simulink model "ANS_GFM_short_term"  (R2021b)
settings: Solver=FixedStepAuto  StartTime=0.0  StopTime=5  FixedStep=Ts  MaxStep=1e-5  RelTol=1e-3
values from neighbouring files (symbols this model uses):
  angle_load = angle(LF.bus(ind_l).Vbus)*180/pi    [init_ANS_GFM_long_term.m]    (also in init_ANS_GFM_short_term.m)
  angleV_LF = Vangle_init/180*pi    [init_ANS_GFM_long_term.m]    (also in init_ANS_GFM_short_term.m)
  awu = 1    [init_ANS_GFM_long_term.m]    (also in init_ANS_GFM_short_term.m)
  C_dc = 1/(Xcdc_pu_or*Zbase_dc_new*100*pi)    [init_ANS_GFM_long_term.m]    (also in init_ANS_GFM_short_term.m)
  C_f = 1/(Xcf_pu_or*Zbase_new*100*pi)    (= 0.013712)    [init_ANS_GFM_long_term.m]    (also in init_ANS_GFM_short_term.m = 0.0141333333333)
  control = 3    [init_ANS_GFM_long_term.m]    (also in init_ANS_GFM_short_term.m = 1)
  D_p = (1/(m_p*w_b))    (= 5209935.26289)    [init_ANS_GFM_long_term.m]    (also in init_ANS_GFM_short_term.m = 5370022.73304)
  Egrid_tmp = 1.054080675694902*400e3    (= 421632.270278)    [init_ANS_GFM_long_term.m]    (also in init_ANS_GFM_short_term.m)
  epsi = 1e-4    (= 0.0001)    [init_ANS_GFM_long_term.m]    (also in init_ANS_GFM_short_term.m)
  eta = m_p*V_m^2    [init_ANS_GFM_long_term.m]    (also in init_ANS_GFM_short_term.m)
  gamma = 2.3    [init_ANS_GFM_long_term.m]    (also in init_ANS_GFM_short_term.m)
  I0_init = [I0_init_a, I0_init_b, I0_init_c]    [init_ANS_GFM_long_term.m]    (also in init_ANS_GFM_short_term.m)
  I_bc = S_bc / (V_bc*sqrt(3))    [init_ANS_GFM_long_term.m]    (also in init_ANS_GFM_short_term.m)
  I_d_int_init = (U_d_int + I_q_int*L_f*w_b - V_d_int - I_d_int*R_f*0)    [init_ANS_GFM_long_term.m]    (also in init_ANS_GFM_short_term.m)
  I_init = [I_init_a, I_init_b, I_init_c]    [init_ANS_GFM_long_term.m]    (also in init_ANS_GFM_short_term.m)
  i_ll = -1.15*(S_bc/Vdc_n)-i_loss_dc    [init_ANS_GFM_long_term.m]    (also in init_ANS_GFM_short_term.m)
  I_max_sat_pu = 1.0 * I_bc *sqrt(2)    [init_ANS_GFM_long_term.m]    (also in init_ANS_GFM_short_term.m)
  I_q_int_init = (U_q_int - I_d_int*L_f*w_b - V_q_int - I_q_int*R_f*0)    [init_ANS_GFM_long_term.m]    (also in init_ANS_GFM_short_term.m)
  i_ul = 1.15*(S_bc/Vdc_n)+i_loss_dc    [init_ANS_GFM_long_term.m]    (also in init_ANS_GFM_short_term.m)
  idppu = 0.95    [init_ANS_GFM_long_term.m]    (also in init_ANS_GFM_short_term.m = 0.92)
  init_dP = -inv(A_pm)*B_pm*dP    [init_ANS_GFM_long_term.m]    (also in init_ANS_GFM_short_term.m)
  init_pm = -inv(A_pm)*B_pm*P_aft    [init_ANS_GFM_long_term.m]    (also in init_ANS_GFM_short_term.m)
  init_tau = -inv(A_tau)*B_tau*idc    [init_ANS_GFM_long_term.m]    (also in init_ANS_GFM_short_term.m)
  J = D_p*tau_f    (= 104198.705258)    [init_ANS_GFM_long_term.m]    (also in init_ANS_GFM_short_term.m = 107400.454661)
  k_dc = eta_1/(Vdc_n*m_p)    [init_ANS_GFM_long_term.m]    (also in init_ANS_GFM_short_term.m)
  K_p = (1/Vdc_n)    [init_ANS_GFM_long_term.m]    (also in init_ANS_GFM_short_term.m)
  K_r = 1/R_dc    [init_ANS_GFM_long_term.m]    (also in init_ANS_GFM_short_term.m)
  Kff_i = 1    [init_ANS_GFM_long_term.m]    (also in init_ANS_GFM_short_term.m)
  Kff_v = 1    [init_ANS_GFM_long_term.m]    (also in init_ANS_GFM_short_term.m)
  Ki_i = (1/n)*1.19    (= 0.0520711785298)    [init_ANS_GFM_long_term.m]    (also in init_ANS_GFM_short_term.m = 0.0505188679245)
  Ki_pll = 4255.3    [init_ANS_GFM_long_term.m]    (also in init_ANS_GFM_short_term.m)
  Ki_v = (n)*1.161022    (= 26.5332227733)    [init_ANS_GFM_long_term.m]    (also in init_ANS_GFM_short_term.m = 27.3485182222)
  ki_v_ac = 2*0.25    (= 0.5)    [init_ANS_GFM_long_term.m]    (also in init_ANS_GFM_short_term.m)
  Kp_i = 0.738891/n    (= 0.032331869895)    [init_ANS_GFM_long_term.m]    (also in init_ANS_GFM_short_term.m = 0.0313680141509)
  Kp_pll = 92    [init_ANS_GFM_long_term.m]    (also in init_ANS_GFM_short_term.m)
  Kp_v = 0.52*n    (= 11.8837333333)    [init_ANS_GFM_long_term.m]    (also in init_ANS_GFM_short_term.m = 12.2488888889)
  kp_v_ac = 0.001    [init_ANS_GFM_long_term.m]    (also in init_ANS_GFM_short_term.m)
  Kpl = 5.0    (= 5)    [init_ANS_GFM_long_term.m]    (also in init_ANS_GFM_short_term.m)
  L1 = cf/sqrt(1+RX^2)*(400e3)^2/Skss/(100*pi)    [init_ANS_GFM_long_term.m]    (also in init_ANS_GFM_short_term.m)
  L_f = Xlf_pu_or*Zbase_new/100/pi    (= 4.37572928821e-06)    [init_ANS_GFM_long_term.m]    (also in init_ANS_GFM_short_term.m = 4.24528301887e-06)
  Lf = 1e6/100/pi    (= 3183.09886184)    [init_ANS_GFM_long_term.m]    (also in init_ANS_GFM_short_term.m = 0.0636619772368)
  m_p = (2*pi*0.5)/(S_bc)    (= 6.10967066042e-10)    [init_ANS_GFM_long_term.m]    (also in init_ANS_GFM_short_term.m = 5.92753330866e-10)
  n = 1/Zb    (= 22.8533333333)    [init_ANS_GFM_long_term.m]    (also in init_ANS_GFM_short_term.m = 23.5555555556)
  P_LF_si = P_LF*S_b    [init_ANS_GFM_long_term.m]    (also in init_ANS_GFM_short_term.m)
  ps = 4440e6/S_bc    (= 0.863477246208)    [init_ANS_GFM_long_term.m]    (also in init_ANS_GFM_short_term.m = 0.837735849057)
  Q_LF_si = Q_LF*S_b    [init_ANS_GFM_long_term.m]    (also in init_ANS_GFM_short_term.m)
  qs = Q_LF*S_b/S_bc    [init_ANS_GFM_long_term.m]    (also in init_ANS_GFM_short_term.m)
  R1 = RX*cf/sqrt(1+RX^2)*(400e3)^2/Skss    [init_ANS_GFM_long_term.m]    (also in init_ANS_GFM_short_term.m)
  R_dc = Rdc_pu_or*Zbase_dc_new    [init_ANS_GFM_long_term.m]    (also in init_ANS_GFM_short_term.m)
  R_f = Rf_pu_or*Zbase_new    (= 2.18786464411e-05)    [init_ANS_GFM_long_term.m]    (also in init_ANS_GFM_short_term.m = 2.12264150943e-05)
  Rf = 1e6    (= 1000000)    [init_ANS_GFM_long_term.m]    (also in init_ANS_GFM_short_term.m = 20)
  S_bc = 5142e6    (= 5142000000)    [init_ANS_GFM_long_term.m]    (also in init_ANS_GFM_short_term.m = 5300000000)
  sat_select = 3    [init_ANS_GFM_long_term.m]    (also in init_ANS_GFM_short_term.m)
  SECM = 3    [init_ANS_GFM_long_term.m]    (also in init_ANS_GFM_short_term.m = 1)
  share_i_load = 1.0    (= 1)    [init_ANS_GFM_long_term.m]    (also in init_ANS_GFM_short_term.m)
  T_en = -0.5    [init_ANS_GFM_long_term.m]    (also in init_ANS_GFM_short_term.m)
  T_off = T_on + 0.1    (= 0.2)    [init_ANS_GFM_long_term.m]    (also in init_ANS_GFM_short_term.m)
  T_on = 0.1    [init_ANS_GFM_long_term.m]    (also in init_ANS_GFM_short_term.m)
  Ts = 2e-6    (= 2e-06)    [init_ANS_GFM_long_term.m]    (also in init_ANS_GFM_short_term.m = 1e-06)
  U_init = [Umag_init_a, Umag_init_b, Umag_init_c]    [init_ANS_GFM_long_term.m]    (also in init_ANS_GFM_short_term.m)
  Uangle_init = angle(V_LF_VSC)*180/pi    [init_ANS_GFM_long_term.m]    (also in init_ANS_GFM_short_term.m)
  Umag_init = abs(V_LF_VSC)*V_bc*sqrt(2/3)    [init_ANS_GFM_long_term.m]    (also in init_ANS_GFM_short_term.m)
  V1_rms = 15e3    (= 15000)    [init_ANS_GFM_long_term.m]    (also in init_ANS_GFM_short_term.m)
  V_d_int = abs(V_LF)*V_bc*sqrt(2/3)    [init_ANS_GFM_long_term.m]    (also in init_ANS_GFM_short_term.m)
  V_d_int_init = (I_d_int + V_q_int*C_f*w_b - I0_d_int)    [init_ANS_GFM_long_term.m]    (also in init_ANS_GFM_short_term.m)
  V_init = [V_init_a, V_init_b, V_init_c]    [init_ANS_GFM_long_term.m]    (also in init_ANS_GFM_short_term.m)
  V_m = sqrt(2/3)*V_bc    [init_ANS_GFM_long_term.m]    (also in init_ANS_GFM_short_term.m)
  V_q_int_init = (I_q_int - V_d_int*C_f*w_b - I0_q_int)    [init_ANS_GFM_long_term.m]    (also in init_ANS_GFM_short_term.m)
  Vdc_n = 3*V_m    [init_ANS_GFM_long_term.m]    (also in init_ANS_GFM_short_term.m)
  Vref = V_LF_mag*V_m    [init_ANS_GFM_long_term.m]    (also in init_ANS_GFM_short_term.m)
  w_b = 2*pi*f_b    (= 314.159265359)    [init_ANS_GFM_long_term.m]    (also in init_ANS_GFM_short_term.m)
  w_f = 2*pi*5    (= 31.4159265359)    [init_ANS_GFM_long_term.m]    (also in init_ANS_GFM_short_term.m)
  Zbase_new = V1_rms^2/S_bc    (= 0.0437572928821)    [init_ANS_GFM_long_term.m]    (also in init_ANS_GFM_short_term.m = 0.0424528301887)
undefined symbols (not defined in the file or in its folder): A_pm, A_tau, B_pm, B_tau, C_pm, C_tau, D_pm, D_tau, find_system, idq0_init, Pm, sm_init, v_d, v_q, Ve
libraries: spsBreakerLib x270, spsGroundLib x21, spsThreePhaseSeriesRLCBranchLib x12, spsabctodq0Lib x11, simulink x9, spsEdgeDetectorLib x8, spsThreePhaseVIMeasurementLib x7, spsLoadFlowBusLib x7, spsSeriesRLCBranchLib x6, spsControlledVoltageSourceLib x6, spsCurrentMeasurementLib x6, spsVoltageMeasurementLib x6
(part 2 of 7)

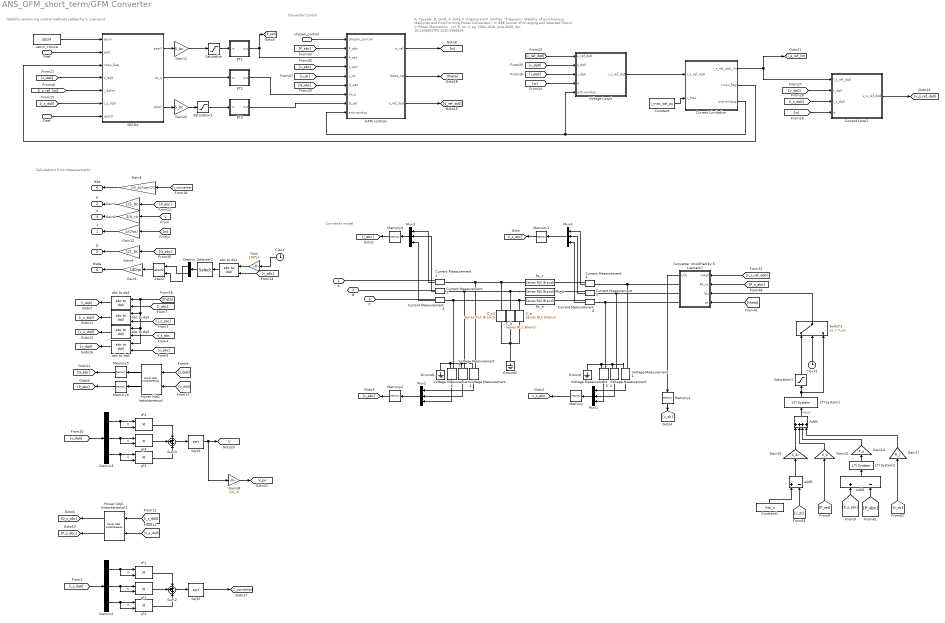
== system ANS_GFM_short_term/GFM Converter ==
  note: A. Tayyebi, D. Groß, A. Anta, F. Kupzog and F. Dörfler, "Frequency Stability of Synchronous Machines and Grid-Forming Power Converters," in IEEE Journal of Emerging and Selected Topics in Power Electronics , vol. 8, no. 2, pp. 1004-1018, June 2020, doi: 10.1109/JESTPE.2020.2966524.
  note: Calculations from Measurements
  note: Converter Control
  note: Stability-enhancing control methods (added by S. Liemann)
  note: Converter model
  chosen_control : Inport
  Pset : Inport  Port=2
  Qset : Inport  Port=3
  Add2 : Sum  Inputs=+-
  Add4 : Sum  Inputs=++++
  Add6 : Sum  Inputs=+-
  Atan2 : Trigonometry  Operator=atan2
  C_a : spsSeriesRLCBranchLib/Series RLC Branch  LConnTagsString=__new0  RConnTagsString=__new0  BranchType=C  Resistance=1  Inductance=1e-3  SetiL0=off  InitialCurrent=0  Capacitance=C_f  Setx0=on  InitialVoltage=V_init_c  Measurements=None
  C_b : spsSeriesRLCBranchLib/Series RLC Branch  LConnTagsString=__new0  RConnTagsString=__new0  BranchType=C  Resistance=1  Inductance=1e-3  SetiL0=off  InitialCurrent=0  Capacitance=C_f  Setx0=on  InitialVoltage=V_init_b  Measurements=None
  C_c1 : spsSeriesRLCBranchLib/Series RLC Branch  LConnTagsString=__new0  RConnTagsString=__new0  BranchType=C  Resistance=1  Inductance=1e-3  SetiL0=off  InitialCurrent=0  Capacitance=C_f  Setx0=on  InitialVoltage=V_init_a  Measurements=None
  Clock : Clock
  Clock1 : Clock
  Constant : Constant  Value=I_max_sat_pu
  Constant1 : Constant  Value=Vdc_n
  Converter (modified by S. Liemann) : Subsystem
  Current Limitation : Subsystem
  Current Loop1 : Subsystem
  Current Measurement{1..6} (6 alike) : spsCurrentMeasurementLib/Current Measurement  PhasorSimulation=off  OutputType=Complex  PSBequivalent=0
  Demux : Demux  Outputs=2
  Demux2 : Demux  Outputs=3
  Demux3 : Demux  Outputs=3
  GFM controls : Subsystem
  Gain : Gain  Gain=100*pi
  Gain1 : Gain  Gain=180/pi
  Gain11 : Gain  Gain=S_bc
  Gain12 : Gain  Gain=1/(2*pi)
  Gain13 : Gain  Gain=K_p
  Gain14 : Gain  Gain=K_p
  Gain16 : Gain  Gain=k_dc
  Gain17 : Gain  Gain=K_r
  Gain18 : Gain  Gain=1/V_m
  Gain22 : Gain  Gain=S_bc
  Gain3 : Gain  Gain=1/(I_bc*sqrt(2))
  Gain4 : Gain  Gain=1/S_bc
  Gain6 : Gain  Gain=1/V_m
  Gain7 : Gain  Gain=1/S_bc
  Ground : spsGroundLib/Ground  LConnTagsString=a
  Ground1 : spsGroundLib/Ground  LConnTagsString=a
  Ground2 : spsGroundLib/Ground  LConnTagsString=a
  LTI System1 : cstblocks/LTI System  sys=ss(A_tau,B_tau,C_tau,D_tau)  IC=[init_tau]
  LTI System2 : cstblocks/LTI System  sys=ss(A_pm,B_pm,C_pm,D_pm)  IC=[init_dP]
  Memory : Memory  InitialCondition=U_init
  Memory1 : Memory  InitialCondition=I_init
  Memory2 : Memory  InitialCondition=V_init
  Memory3 : Memory  InitialCondition=I0_init
  Memory4 : Memory  InitialCondition=Vdc_n
  Memory5 : Memory  InitialCondition=Q_LF_si
  Memory6 : Memory  InitialCondition=P_LF_si
  Mux{1..4} (4 alike) : Mux  Inputs=3
  PT1 : Subsystem
  PT2 : Subsystem
  PT3 : Subsystem
  "Power (dq0, Instantaneous)" : spsPowerdq0InstantaneousLib/Power (dq0, Instantaneous)
      settings: SourceProductBaseCode=PS
  "Power (dq0, Instantaneous)1" : spsPowerdq0InstantaneousLib/Power (dq0, Instantaneous)
      settings: SourceProductBaseCode=PS
  RL_a : spsSeriesRLCBranchLib/Series RLC Branch  LConnTagsString=__new0  RConnTagsString=__new0  BranchType=RL  Resistance=R_f  Inductance=L_f  SetiL0=on  InitialCurrent=I_init_c  Capacitance=1e-6  Setx0=off  InitialVoltage=0  Measurements=Branch voltage and current
  RL_b : spsSeriesRLCBranchLib/Series RLC Branch  LConnTagsString=__new0  RConnTagsString=__new0  BranchType=RL  Resistance=R_f  Inductance=L_f  SetiL0=on  InitialCurrent=I_init_b  Capacitance=1e-6  Setx0=off  InitialVoltage=0  Measurements=None
  RL_c : spsSeriesRLCBranchLib/Series RLC Branch  LConnTagsString=__new0  RConnTagsString=__new0  BranchType=RL  Resistance=R_f  Inductance=L_f  SetiL0=on  InitialCurrent=I_init_a  Capacitance=1e-6  Setx0=off  InitialVoltage=0  Measurements=None
  SECMs : Subsystem
  Saturation : Saturate  UpperLimit=S_bc  LowerLimit=-S_bc
  Saturation1 : Saturate  UpperLimit=i_ul  LowerLimit=i_ll
  Saturation2 : Saturate  UpperLimit=S_bc  LowerLimit=-S_bc
  Selector2 : Selector  InputPortWidth=3  IndexOptions=Index vector (dialog)  Indices=[1 2]  OutputSizes=1
  Sqrt2 : Sqrt  SaturateOnIntegerOverflow=on
  Sqrt3 : Sqrt  SaturateOnIntegerOverflow=on
  Sum2 : Sum  Inputs=+++  InputSameDT=on  SaturateOnIntegerOverflow=on  OutDataTypeStr=Inherit: Same as first input
  Sum3 : Sum  Inputs=+++  InputSameDT=on  SaturateOnIntegerOverflow=on  OutDataTypeStr=Inherit: Same as first input
  Switch1 : Switch  Criteria=u2 > Threshold  Threshold=T_en
  Voltage Loop1 : Subsystem
  Voltage Measurement{1..6} (6 alike) : spsVoltageMeasurementLib/Voltage Measurement  PhasorSimulation=off  OutputType=Complex  PSBequivalent=0
  abc to dq{1,3..6} (5 alike) : spsabctodq0Lib/abc to dq0  Alignment=90 degrees behind phase A axis
  d²1 : Product  InputSameDT=on  RndMeth=Zero  SaturateOnIntegerOverflow=on  OutDataTypeStr=Inherit: Same as first input
  d²2 : Product  InputSameDT=on  RndMeth=Zero  SaturateOnIntegerOverflow=on  OutDataTypeStr=Inherit: Same as first input
  q²{1..2,4..5} (4 alike) : Product  InputSameDT=on  RndMeth=Zero  SaturateOnIntegerOverflow=on  OutDataTypeStr=Inherit: Same as first input
  secm_choice : Constant  Value=SECM
  A : PMIOPort  Side=Right
  B : PMIOPort  Port=2  Side=Right
  C : PMIOPort  Port=3  Side=Right
  f : Outport  VectorParamsAs1DForOutWhenUnconnected=off
  P : Outport  Port=2  VectorParamsAs1DForOutWhenUnconnected=off
  V : Outport  Port=3  VectorParamsAs1DForOutWhenUnconnected=off
  Iabs : Outport  Port=4  VectorParamsAs1DForOutWhenUnconnected=off
  Q : Outport  Port=5  VectorParamsAs1DForOutWhenUnconnected=off
  theta : Outport  Port=6  VectorParamsAs1DForOutWhenUnconnected=off
  tag scope: V=global, V_pu=global, v_s_abc=global
  wires:
  [i_s_dq0] -> "Power (dq0, Instantaneous)1"/2
  Voltage Measurement5/1 -> Mux2/2
  [v_s_dq0] -> "Power (dq0, Instantaneous)1"/1
  Voltage Measurement3/1 -> Mux1/3
  Voltage Measurement1/1 -> Mux1/1
  Memory1/1 -> [i_s_abc]
  q²1/1 -> Sum2/2
  Current Measurement4/1 -> Mux4/1
  Mux3/1 -> Memory3/1
  Constant1/1 -> Add6/1
  Voltage Measurement4/1 -> Mux2/1
  [I_converter] -> Gain3/1
  LTI System1/1 -> Saturation1/1, Switch1/3
  Memory2/1 -> [v_abc]
  Memory/1 -> [v_s_abc]
  Sum2/1 -> Sqrt2/1
  Demux2/2 -> q²1/2, q²1/1  "q"
  Add6/1 -> Gain16/1
  [v_dq0] -> "Power (dq0, Instantaneous)"/1
  Current Measurement5/1 -> Mux4/2
  Gain3/1 -> Iabs/1
  [i_s_dq0] -> Demux2/1
  [theta] -> abc to dq3/2, abc to dq6/2, abc to dq5/2, abc to dq4/2
  d²1/1 -> Sum2/1
  [P_abc] -> Gain7/1
  Voltage Measurement2/1 -> Mux1/2
  [P_s_abc] -> Add2/1
  Demux2/3 -> q²2/2, q²2/1  "0"
  Gain16/1 -> Add4/1
  Gain13/1 -> Add4/2
  Demux3/2 -> q²4/2, q²4/1  "q"
  "Power (dq0, Instantaneous)1"/2 -> [Q_s_abc]
  Sqrt3/1 -> Gain18/1, [V]
  [P_abc] -> Add2/2
  Saturation1/1 -> Switch1/1
  [v_dc] -> Add6/2
  Demux3/1 -> d²2/2, d²2/1  "d"
  Demux2/1 -> d²1/2, d²1/1  "d"
  [i_abc] -> abc to dq3/1
  Clock1/1 -> Switch1/2
  Current Measurement1/1 -> Mux3/1
  [P_set] -> Gain13/1
  abc to dq4/1 -> [i_s_dq0]
  Add4/1 -> LTI System1/1  "input"
  Current Measurement3/1 -> Mux3/3
  [v_dq0] -> Demux3/1
  Add2/1 -> LTI System2/1
  abc to dq3/1 -> [i_dq0]
  Current Measurement6/1 -> Mux4/3
  Voltage Measurement6/1 -> Mux2/3
  Mux1/1 -> Memory/1
  [v_dc] -> Gain17/1
  [w] -> Gain12/1
  [i_dq0] -> "Power (dq0, Instantaneous)"/2
  Gain12/1 -> f/1
  Gain7/1 -> P/1
  Current Measurement2/1 -> Mux3/2
  [i_s_abc] -> abc to dq4/1
  q²4/1 -> Sum3/2
  Mux2/1 -> Memory2/1
  abc to dq6/1 -> [v_dq0]
  [v_abc] -> abc to dq6/1
  Gain6/1 -> V/1
  [v_s_abc] -> abc to dq5/1
  q²5/1 -> Sum3/3
  Memory3/1 -> [i_abc]
  Memory4/1 -> [v_dc]
  [V] -> Gain6/1
  d²2/1 -> Sum3/1
  Sum3/1 -> Sqrt3/1
  Switch1/1 -> Converter (modified by S. Liemann)/3(Idc)
  q²2/1 -> Sum2/3
  Demux3/3 -> q²5/2, q²5/1  "0"
  Current Limitation/1(i_s_ref_dq0_lim) -> Current Loop1/1(i_s_ref_dq0), [i_s_ref_lim]
  Voltage Loop1/1(i_s_ref_dq0) -> Current Limitation/1(i_s_ref_dq0)
  [i_s_dq0] -> Current Loop1/3(i_s_dq0)
  Current Limitation/3(anti-windup) -> Voltage Loop1/5(anti-windup), GFM controls/9(anti-windup)
  [i_dq0] -> Voltage Loop1/3(i_dq0)
  [w] -> Current Loop1/4(w)
  Constant/1 -> Current Limitation/2(i_max)
  Current Loop1/1(v_s_ref_dq0) -> [v_s_ref_dq0]
  [v_ref_dq0] -> Voltage Loop1/1(v_ref_dq0)
  [v_dq0] -> Current Loop1/2(v_dq0)
  [w] -> Voltage Loop1/4(w)
  Gain4/1 -> Q/1
  [Q_abc] -> Gain4/1
  GFM controls/2(theta_ref) -> [theta]
  GFM controls/3(v_ref_dqo) -> [v_ref_dq0]
  [P_abc] -> GFM controls/2(P_abc)
  PT1/1(out) -> GFM controls/3(P_set), [P_set]
  [v_abc] -> GFM controls/4(v_abc)
  [Q_abc] -> GFM controls/6(Q_abc)
  [v_dc] -> GFM controls/5(v_dc)
  Mux4/1 -> Memory1/1
  [v_dq0] -> Voltage Loop1/2(v_dq0)
  abc to dq5/1 -> [v_s_dq0]
  [v_s_ref_dq0] -> Converter (modified by S. Liemann)/1(Vdq0)
  GFM controls/1(w_ref) -> [w]
  Pset/1 -> SECMs/2(pset)
  [theta] -> Converter (modified by S. Liemann)/4(wt)
  [P_s_abc] -> Converter (modified by S. Liemann)/2(Pe_ac)
  LTI System2/1 -> Gain14/1
  "Power (dq0, Instantaneous)1"/1 -> [P_s_abc]
  "Power (dq0, Instantaneous)"/1 -> Memory6/1
  "Power (dq0, Instantaneous)"/2 -> Memory5/1
  Saturation/1 -> PT1/1(in)
  Memory5/1 -> [Q_abc]
  Memory6/1 -> [P_abc]
  Selector2/1 -> Demux/1
  abc to dq1/1 -> Selector2/1
  Demux/2 -> Atan2/1
  Demux/1 -> Atan2/2
  Atan2/1 -> Gain1/1
  Gain1/1 -> theta/1
  [v_abc] -> abc to dq1/1
  Gain/1 -> abc to dq1/2
  Clock/1 -> Gain/1
  Sqrt2/1 -> [I_converter]
  chosen_control/1 -> GFM controls/1(chosen_control)
  Gain14/1 -> Add4/3
  Gain17/1 -> Add4/4
  Converter (modified by S. Liemann)/1(Udc) -> Memory4/1
  Gain18/1 -> [V_pu]
  [i_s_dq0] -> SECMs/6(i_s_dq0)
  secm_choice/1 -> SECMs/1(secm)
  [v_dq0] -> SECMs/4(V_dq0)
  SECMs/1(pset*) -> Gain11/1
  Gain11/1 -> Saturation/1
  SECMs/2(dv_q) -> PT2/1(in)
  PT2/1(out) -> GFM controls/7(dv_q)
  [i_s_ref_lim] -> SECMs/5(i_dqlim)
  Qset/1 -> SECMs/7(qset0)
  PT3/1(out) -> GFM controls/8(Q_set)
  SECMs/3(qset*) -> Gain22/1
  Gain22/1 -> Saturation2/1
  Saturation2/1 -> PT3/1(in)
  Current Limitation/2(imax_flag) -> SECMs/3(imax_flag)
  connections:
  Ground/LConn1 -- Voltage Measurement3/LConn2 -- Voltage Measurement1/LConn2 -- Voltage Measurement2/LConn2
  Voltage Measurement6/LConn1 -- Current Measurement3/LConn1 -- C_a/LConn1 -- RL_a/RConn1
  Voltage Measurement6/LConn2 -- Ground1/LConn1 -- Voltage Measurement4/LConn2 -- Voltage Measurement5/LConn2
  Voltage Measurement2/LConn1 -- Current Measurement5/LConn1 -- Converter (modified by S. Liemann)/RConn2
  Voltage Measurement4/LConn1 -- Current Measurement1/LConn1 -- C_c1/LConn1 -- RL_c/RConn1
  RL_b/RConn1 -- C_b/LConn1 -- Current Measurement2/LConn1 -- Voltage Measurement5/LConn1
  C_b/RConn1 -- C_c1/RConn1 -- Ground2/LConn1 -- C_a/RConn1
  Current Measurement6/LConn1 -- Voltage Measurement3/LConn1 -- Converter (modified by S. Liemann)/RConn3
  Voltage Measurement1/LConn1 -- Current Measurement4/LConn1 -- Converter (modified by S. Liemann)/RConn1
  Current Measurement4/RConn1 -- RL_c/LConn1
  Current Measurement6/RConn1 -- RL_a/LConn1
  Current Measurement5/RConn1 -- RL_b/LConn1
  Current Measurement1/RConn1 -- A/RConn1
  Current Measurement2/RConn1 -- B/RConn1
  Current Measurement3/RConn1 -- C/RConn1

== system ANS_GFM_short_term/HVRT & LVRT ==
  Uin : Inport
  Clock2 : Clock
  Constant5 : Constant  Value=0
  Constant6 : Constant
  Constant7 : Constant  Value=1.3
  Constant8 : Constant  Value=1.2
  Gain5 : Gain  Gain=0.85/2.85
  Integrator : Integrator
  Relational Operator : RelationalOperator  Operator=<  OutDataTypeStr=boolean  RndMeth=Simplest
  Relational Operator1 : RelationalOperator  Operator=>  OutDataTypeStr=boolean  RndMeth=Simplest
  Switch : Switch  Threshold=T_on+0.15
  Switch1 : Switch  Threshold=T_on+3.0
  Switch2 : Switch  Threshold=T_on+0.1
  HVRT-Flag : Outport
  HVRT curve : Outport  Port=2
  LVRT-Flag : Outport  Port=3
  LVRT curve : Outport  Port=4
  wires:
  Constant5/1 -> Switch/3, Switch1/1
  Integrator/1 -> LVRT curve/1, Relational Operator/2
  Switch2/1 -> HVRT curve/1, Relational Operator1/2
  Relational Operator/1 -> LVRT-Flag/1
  Clock2/1 -> Switch2/2, Switch/2, Switch1/2
  Constant6/1 -> Switch/1
  Uin/1 -> Relational Operator1/1, Relational Operator/1
  Switch/1 -> Switch1/3
  Switch1/1 -> Gain5/1
  Gain5/1 -> Integrator/1
  Relational Operator1/1 -> HVRT-Flag/1
  Constant8/1 -> Switch2/1
  Constant7/1 -> Switch2/3

== system ANS_GFM_short_term/OLTC ==
  note: G. Sybille, P. Giroux Hydro-Quebec (IREQ)
  note: This Three-Phase OLTC Regulating Transformer is built with three Multi-Winding Transformer blocks
      | and three On-Load Tap Changers (OLTC) subsystems using switches.
      | It implements a fixed number of taps (8 taps per phase +  tap 0 (nominal voltage ratio)).
      |
      | In order to change the number of taps you must modify the 3 Transformer blocks
      | and the 3  OLTC blocks as explained in the  the procedure given below:
  Vm (pu) : Inport
  " OLTC Control" : Subsystem  mask{NumberOfTaps=NumberOfTaps, TapSelectionTime=TapSelectionTime, TransferTime=TransferTime, InitialTap=InitialTap}
      mask prompts: NumberOfTaps "Number of taps:"; TapSelectionTime "Operating time of the tap selector (typical 3-10 s):"; TransferTime "Operating time of the transfer switch (typical 40-60 ms):"; InitialTap "Initial tap:"
      mask init:
      | TapVector=0:NumberOfTaps;
      | InitialStates=zeros(1,NumberOfTaps+1);
  Constant : Constant  Value=RegulatorOn
  Display : Display  Commented=on
  Goto Tag Visibility : GotoTagVisibility  GotoTag=SwSelect
  Goto Tag Visibility1 : GotoTagVisibility  GotoTag=SwTransfer
  Goto Tag Visibility2 : GotoTagVisibility  GotoTag=SwInversion
  Ground : spsGroundLib/Ground  LConnTagsString=a
  Ground1 : spsGroundLib/Ground  LConnTagsString=a
  Ground2 : spsGroundLib/Ground  LConnTagsString=a
  OLTCA : Subsystem  mask{NumberOfTaps=NumberOfTaps, InitialTap=InitialTap, Rtransfer=Rtransfer}
      mask prompts: NumberOfTaps "Nombre de prises:"; InitialTap "Prise initiale:"; Rtransfer "Resistance de court circuit (ohms):"
      mask init:
      | TapVector=0:NumberOfTaps;
      | InitialStates=zeros(1,NumberOfTaps+1);
      | InitialStates(abs(InitialTap)+1)=1;
      | 
      | InitialStateInv1=(InitialTap>=0);
      | InitialStateInv2=(InitialTap<0);
      | InitialStateInv3=InitialStateInv1;
      | InitialStateInv4=InitialStateInv2;
  OLTCA1 : Subsystem  mask{NumberOfTaps=NumberOfTaps, InitialTap=InitialTap, Rtransfer=Rtransfer}
      mask prompts: NumberOfTaps "Nombre de prises:"; InitialTap "Prise initiale:"; Rtransfer "Resistance de court circuit (ohms):"
      mask init: same as ANS_GFM_short_term/OLTC/OLTCA
  OLTCA2 : Subsystem  mask{NumberOfTaps=NumberOfTaps, InitialTap=InitialTap, Rtransfer=Rtransfer}
      mask prompts: NumberOfTaps "Nombre de prises:"; InitialTap "Prise initiale:"; Rtransfer "Resistance de court circuit (ohms):"
      mask init: same as ANS_GFM_short_term/OLTC/OLTCA
  OLTCA3 : Subsystem  Commented=on  mask{NumberOfTaps=NumberOfTaps, InitialTap=InitialTap, Rtransfer=Rtransfer}
      mask prompts: NumberOfTaps "Nombre de prises:"; InitialTap "Prise initiale:"; Rtransfer "Resistance de court circuit (ohms):"
      mask init: same as ANS_GFM_short_term/OLTC/OLTCA
  OLTCC1 : Subsystem  Commented=on  mask{NumberOfTaps=NumberOfTaps, InitialTap=InitialTap, Rtransfer=Rtransfer}
      mask prompts: NumberOfTaps "Nombre de prises:"; InitialTap "Prise initiale:"; Rtransfer "Resistance de court circuit (ohms):"
      mask init: same as ANS_GFM_short_term/OLTC/OLTCA
  Subsystem : Subsystem
      mask Display: disp('Procedure\n to change\n the number of taps')
  TransformerA : spsMultiWindingTransformerLib/Multi-Winding Transformer  LeftWindings=1  RightWindings=2  TappedWindings=taps on upper right winding  NumberOfTaps=19  SetSaturation=off  Hysteresis=off  DataFile='hysteresis.mat'  Measurements=None  UNITS=pu  NominalPower="[Pnom  Fnom]"  NominalVoltages=[Vnom1 VnomTaps Vnom2 ]  WindingResistances=[Rpu1 RpuTaps Rpu2]  WindingInductances="[Xpu1 XpuTaps  Xpu2 ]"  Rm=Rm  Lm=Lm  Saturation=[ 0,0 ; 0.0024,1.2 ; 1.0,1.52 ]  BreakLoop=off  DiscreteSolver=Trapezoidal iterative  DataType=off  InitialFlux=0  TransfoNumber=1
      settings: SourceProductBaseCode=PS
  TransformerB : spsMultiWindingTransformerLib/Multi-Winding Transformer  LeftWindings=1  RightWindings=2  TappedWindings=taps on upper right winding  NumberOfTaps=19  SetSaturation=off  Hysteresis=off  DataFile='hysteresis.mat'  Measurements=None  UNITS=pu  NominalPower="[Pnom  Fnom]"  NominalVoltages=[Vnom1 VnomTaps Vnom2 ]  WindingResistances=[Rpu1 RpuTaps Rpu2]  WindingInductances="[Xpu1 XpuTaps  Xpu2 ]"  Rm=Rm  Lm=Lm  Saturation=[ 0,0 ; 0.0024,1.2 ; 1.0,1.52 ]  BreakLoop=off  DiscreteSolver=Trapezoidal iterative  DataType=off  InitialFlux=0  TransfoNumber=1
      settings: SourceProductBaseCode=PS
  TransformerC : spsMultiWindingTransformerLib/Multi-Winding Transformer  LeftWindings=1  RightWindings=2  TappedWindings=taps on upper right winding  NumberOfTaps=19  SetSaturation=off  Hysteresis=off  DataFile='hysteresis.mat'  Measurements=None  UNITS=pu  NominalPower="[Pnom  Fnom]"  NominalVoltages=[Vnom1 VnomTaps Vnom2 ]  WindingResistances=[Rpu1 RpuTaps Rpu2]  WindingInductances="[Xpu1 XpuTaps  Xpu2 ]"  Rm=Rm  Lm=Lm  Saturation=[ 0,0 ; 0.0024,1.2 ; 1.0,1.52 ]  BreakLoop=off  DiscreteSolver=Trapezoidal iterative  DataType=off  InitialFlux=0  TransfoNumber=1
      settings: SourceProductBaseCode=PS
  Voltage regulator : Subsystem  mask{Vref=RegulatorVref, DeadBand=RegulatorDeadBand, TimeDelay=RegulatorDelay}
      mask prompts: Vref "Vref (pu)"; DeadBand "Deadband (pu)"; TimeDelay "Time delay (s)"
  A : PMIOPort  Tag=PMCPort  Side=Left
  B : PMIOPort  Tag=PMCPort  Port=2  Side=Left
  C : PMIOPort  Tag=PMCPort  Port=3  Side=Left
  a : PMIOPort  Tag=PMCPort  Port=4  Side=Right
  b : PMIOPort  Tag=PMCPort  Port=5  Side=Right
  c : PMIOPort  Tag=PMCPort  Port=6  Side=Right
  Tap : Outport  VectorParamsAs1DForOutWhenUnconnected=off
  tag scope: SwInversion=scoped, SwSelect=scoped, SwTransfer=scoped
  wires:
  Constant/1 -> Voltage regulator/3(RegOn)
  Vm (pu)/1 -> Voltage regulator/1(Vmes (pu))
  Voltage regulator/2(Down) -> " OLTC Control"/2(Down)
  " OLTC Control"/5(Ready) -> Voltage regulator/2(Ready)
  Voltage regulator/1(Up) -> " OLTC Control"/1(Up)
  " OLTC Control"/4(SwInv) -> [SwInversion]
  " OLTC Control"/1(Tap) -> Display/1, Tap/1  "Tap"
  " OLTC Control"/2(SwSelect) -> [SwSelect]
  " OLTC Control"/3(SwTr) -> [SwTransfer]
  connections:
  OLTCA/RConn22 -- TransformerA/RConn22
  OLTCA/RConn21 -- TransformerA/RConn21
  OLTCA/RConn20 -- TransformerA/RConn20
  OLTCA/RConn19 -- TransformerA/RConn19
  OLTCA/RConn18 -- TransformerA/RConn18
  OLTCA/RConn17 -- TransformerA/RConn17
  OLTCA/RConn16 -- TransformerA/RConn16
  OLTCA/RConn15 -- TransformerA/RConn15
  OLTCA/RConn13 -- TransformerA/RConn13
  OLTCA/RConn12 -- TransformerA/RConn12
  OLTCA/RConn14 -- TransformerA/RConn14
  OLTCA/RConn11 -- TransformerA/RConn11
  OLTCA/RConn10 -- TransformerA/RConn10
  OLTCA/RConn9 -- TransformerA/RConn9
  OLTCA/RConn8 -- TransformerA/RConn8
  OLTCA/RConn7 -- TransformerA/RConn7
  OLTCA/RConn6 -- TransformerA/RConn6
  OLTCA/RConn5 -- TransformerA/RConn5
  OLTCA/RConn4 -- TransformerA/RConn4
  OLTCA/RConn3 -- TransformerA/RConn3
  OLTCA/RConn2 -- TransformerA/RConn2
  OLTCA/RConn1 -- TransformerA/RConn1
  Ground/LConn1 -- TransformerA/RConn23
  OLTCA/LConn1 -- a/RConn1
  Ground1/LConn1 -- TransformerB/RConn23
  OLTCA1/RConn7 -- TransformerB/RConn7
  OLTCA1/RConn17 -- TransformerB/RConn17
  OLTCA1/RConn21 -- TransformerB/RConn21
  OLTCA1/RConn15 -- TransformerB/RConn15
  OLTCA1/RConn14 -- TransformerB/RConn14
  OLTCA1/RConn3 -- TransformerB/RConn3
  OLTCA1/RConn9 -- TransformerB/RConn9
  OLTCA1/RConn13 -- TransformerB/RConn13
  OLTCA1/RConn8 -- TransformerB/RConn8
  OLTCA1/RConn1 -- TransformerB/RConn1
  OLTCA1/RConn16 -- TransformerB/RConn16
  OLTCA1/RConn12 -- TransformerB/RConn12
  OLTCA1/RConn4 -- TransformerB/RConn4
  OLTCA1/RConn5 -- TransformerB/RConn5
  OLTCA1/RConn2 -- TransformerB/RConn2
  OLTCA1/RConn10 -- TransformerB/RConn10
  OLTCA1/RConn6 -- TransformerB/RConn6
  OLTCA1/RConn20 -- TransformerB/RConn20
  OLTCA1/RConn22 -- TransformerB/RConn22
  OLTCA1/RConn18 -- TransformerB/RConn18
  OLTCA1/RConn19 -- TransformerB/RConn19
  OLTCA1/RConn11 -- TransformerB/RConn11
  Ground2/LConn1 -- TransformerC/RConn23
  OLTCA2/RConn7 -- TransformerC/RConn7
  OLTCA2/RConn17 -- TransformerC/RConn17
  OLTCA2/RConn21 -- TransformerC/RConn21
  OLTCA2/RConn15 -- TransformerC/RConn15
  OLTCA2/RConn14 -- TransformerC/RConn14
  OLTCA2/RConn3 -- TransformerC/RConn3
  OLTCA2/RConn9 -- TransformerC/RConn9
  OLTCA2/RConn13 -- TransformerC/RConn13
  OLTCA2/RConn8 -- TransformerC/RConn8
  OLTCA2/RConn1 -- TransformerC/RConn1
  OLTCA2/RConn16 -- TransformerC/RConn16
  OLTCA2/RConn12 -- TransformerC/RConn12
  OLTCA2/RConn4 -- TransformerC/RConn4
  OLTCA2/RConn5 -- TransformerC/RConn5
  OLTCA2/RConn2 -- TransformerC/RConn2
  OLTCA2/RConn10 -- TransformerC/RConn10
  OLTCA2/RConn6 -- TransformerC/RConn6
  OLTCA2/RConn20 -- TransformerC/RConn20
  OLTCA2/RConn22 -- TransformerC/RConn22
  OLTCA2/RConn18 -- TransformerC/RConn18
  OLTCA2/RConn19 -- TransformerC/RConn19
  OLTCA2/RConn11 -- TransformerC/RConn11
  OLTCA2/LConn1 -- c/RConn1
  OLTCA1/LConn1 -- b/RConn1
  TransformerA/LConn2 -- TransformerB/LConn1 -- B/RConn1
  TransformerB/LConn2 -- C/RConn1 -- TransformerC/LConn1
  TransformerC/LConn2 -- A/RConn1 -- TransformerA/LConn1

== system ANS_GFM_short_term/OLTC for load flow ==
  note: G. Sybille, P. Giroux Hydro-Quebec (IREQ)
  note: This Three-Phase OLTC Regulating Transformer is built with three Multi-Winding Transformer blocks
      | and three On-Load Tap Changers (OLTC) subsystems using switches.
      | It implements a fixed number of taps (8 taps per phase +  tap 0 (nominal voltage ratio)).
      |
      | In order to change the number of taps you must modify the 3 Transformer blocks
      | and the 3  OLTC blocks as explained in the  the procedure given below:
  Vm (pu) : Inport
  " OLTC Control" : Subsystem  mask{NumberOfTaps=NumberOfTaps, TapSelectionTime=TapSelectionTime, TransferTime=TransferTime, InitialTap=InitialTap}
      mask prompts: NumberOfTaps "Number of taps:"; TapSelectionTime "Operating time of the tap selector (typical 3-10 s):"; TransferTime "Operating time of the transfer switch (typical 40-60 ms):"; InitialTap "Initial tap:"
      mask init:
      | TapVector=0:NumberOfTaps;
      | InitialStates=zeros(1,NumberOfTaps+1);
  Constant : Constant  Value=RegulatorOn
  Display : Display  Commented=on
  Goto Tag Visibility : GotoTagVisibility  GotoTag=SwSelect
  Goto Tag Visibility1 : GotoTagVisibility  GotoTag=SwTransfer
  Goto Tag Visibility2 : GotoTagVisibility  GotoTag=SwInversion
  Ground : spsGroundLib/Ground  LConnTagsString=a
  Ground1 : spsGroundLib/Ground  LConnTagsString=a
  Ground2 : spsGroundLib/Ground  LConnTagsString=a
  OLTCA : Subsystem  mask{NumberOfTaps=NumberOfTaps, InitialTap=InitialTap, Rtransfer=Rtransfer}
      mask prompts: NumberOfTaps "Nombre de prises:"; InitialTap "Prise initiale:"; Rtransfer "Resistance de court circuit (ohms):"
      mask init: same as ANS_GFM_short_term/OLTC/OLTCA
  OLTCA1 : Subsystem  mask{NumberOfTaps=NumberOfTaps, InitialTap=InitialTap, Rtransfer=Rtransfer}
      mask prompts: NumberOfTaps "Nombre de prises:"; InitialTap "Prise initiale:"; Rtransfer "Resistance de court circuit (ohms):"
      mask init: same as ANS_GFM_short_term/OLTC/OLTCA
  OLTCA2 : Subsystem  mask{NumberOfTaps=NumberOfTaps, InitialTap=InitialTap, Rtransfer=Rtransfer}
      mask prompts: NumberOfTaps "Nombre de prises:"; InitialTap "Prise initiale:"; Rtransfer "Resistance de court circuit (ohms):"
      mask init: same as ANS_GFM_short_term/OLTC/OLTCA
  OLTCA3 : Subsystem  Commented=on  mask{NumberOfTaps=NumberOfTaps, InitialTap=InitialTap, Rtransfer=Rtransfer}
      mask prompts: NumberOfTaps "Nombre de prises:"; InitialTap "Prise initiale:"; Rtransfer "Resistance de court circuit (ohms):"
      mask init: same as ANS_GFM_short_term/OLTC/OLTCA
  OLTCC1 : Subsystem  Commented=on  mask{NumberOfTaps=NumberOfTaps, InitialTap=InitialTap, Rtransfer=Rtransfer}
      mask prompts: NumberOfTaps "Nombre de prises:"; InitialTap "Prise initiale:"; Rtransfer "Resistance de court circuit (ohms):"
      mask init: same as ANS_GFM_short_term/OLTC/OLTCA
  Subsystem : Subsystem
      mask Display: disp('Procedure\n to change\n the number of taps')
  TransformerA : spsMultiWindingTransformerLib/Multi-Winding Transformer  LeftWindings=1  RightWindings=2  TappedWindings=taps on upper right winding  NumberOfTaps=19  SetSaturation=off  Hysteresis=off  DataFile='hysteresis.mat'  Measurements=None  UNITS=pu  NominalPower="[Pnom  Fnom]"  NominalVoltages=[Vnom1 VnomTaps Vnom2 ]  WindingResistances=[Rpu1 RpuTaps Rpu2]  WindingInductances="[Xpu1 XpuTaps  Xpu2 ]"  Rm=Rm  Lm=Lm  Saturation=[ 0,0 ; 0.0024,1.2 ; 1.0,1.52 ]  BreakLoop=off  DiscreteSolver=Trapezoidal iterative  DataType=off  InitialFlux=0  TransfoNumber=1
      settings: SourceProductBaseCode=PS
  TransformerB : spsMultiWindingTransformerLib/Multi-Winding Transformer  LeftWindings=1  RightWindings=2  TappedWindings=taps on upper right winding  NumberOfTaps=19  SetSaturation=off  Hysteresis=off  DataFile='hysteresis.mat'  Measurements=None  UNITS=pu  NominalPower="[Pnom  Fnom]"  NominalVoltages=[Vnom1 VnomTaps Vnom2 ]  WindingResistances=[Rpu1 RpuTaps Rpu2]  WindingInductances="[Xpu1 XpuTaps  Xpu2 ]"  Rm=Rm  Lm=Lm  Saturation=[ 0,0 ; 0.0024,1.2 ; 1.0,1.52 ]  BreakLoop=off  DiscreteSolver=Trapezoidal iterative  DataType=off  InitialFlux=0  TransfoNumber=1
      settings: SourceProductBaseCode=PS
  TransformerC : spsMultiWindingTransformerLib/Multi-Winding Transformer  LeftWindings=1  RightWindings=2  TappedWindings=taps on upper right winding  NumberOfTaps=19  SetSaturation=off  Hysteresis=off  DataFile='hysteresis.mat'  Measurements=None  UNITS=pu  NominalPower="[Pnom  Fnom]"  NominalVoltages=[Vnom1 VnomTaps Vnom2 ]  WindingResistances=[Rpu1 RpuTaps Rpu2]  WindingInductances="[Xpu1 XpuTaps  Xpu2 ]"  Rm=Rm  Lm=Lm  Saturation=[ 0,0 ; 0.0024,1.2 ; 1.0,1.52 ]  BreakLoop=off  DiscreteSolver=Trapezoidal iterative  DataType=off  InitialFlux=0  TransfoNumber=1
      settings: SourceProductBaseCode=PS
  Voltage regulator : Subsystem  mask{Vref=RegulatorVref, DeadBand=RegulatorDeadBand, TimeDelay=RegulatorDelay}
      mask prompts: Vref "Vref (pu)"; DeadBand "Deadband (pu)"; TimeDelay "Time delay (s)"
  A : PMIOPort  Tag=PMCPort  Side=Left
  B : PMIOPort  Tag=PMCPort  Port=2  Side=Left
  C : PMIOPort  Tag=PMCPort  Port=3  Side=Left
  a : PMIOPort  Tag=PMCPort  Port=4  Side=Right
  b : PMIOPort  Tag=PMCPort  Port=5  Side=Right
  c : PMIOPort  Tag=PMCPort  Port=6  Side=Right
  Tap : Outport  VectorParamsAs1DForOutWhenUnconnected=off
  tag scope: SwInversion=scoped, SwSelect=scoped, SwTransfer=scoped
  wires:
  Constant/1 -> Voltage regulator/3(RegOn)
  Vm (pu)/1 -> Voltage regulator/1(Vmes (pu))
  Voltage regulator/2(Down) -> " OLTC Control"/2(Down)
  " OLTC Control"/5(Ready) -> Voltage regulator/2(Ready)
  Voltage regulator/1(Up) -> " OLTC Control"/1(Up)
  " OLTC Control"/4(SwInv) -> [SwInversion]
  " OLTC Control"/1(Tap) -> Display/1, Tap/1  "Tap"
  " OLTC Control"/2(SwSelect) -> [SwSelect]
  " OLTC Control"/3(SwTr) -> [SwTransfer]
  connections:
  OLTCA/RConn22 -- TransformerA/RConn22
  OLTCA/RConn21 -- TransformerA/RConn21
  OLTCA/RConn20 -- TransformerA/RConn20
  OLTCA/RConn19 -- TransformerA/RConn19
  OLTCA/RConn18 -- TransformerA/RConn18
  OLTCA/RConn17 -- TransformerA/RConn17
  OLTCA/RConn16 -- TransformerA/RConn16
  OLTCA/RConn15 -- TransformerA/RConn15
  OLTCA/RConn13 -- TransformerA/RConn13
  OLTCA/RConn12 -- TransformerA/RConn12
  OLTCA/RConn14 -- TransformerA/RConn14
  OLTCA/RConn11 -- TransformerA/RConn11
  OLTCA/RConn10 -- TransformerA/RConn10
  OLTCA/RConn9 -- TransformerA/RConn9
  OLTCA/RConn8 -- TransformerA/RConn8
  OLTCA/RConn7 -- TransformerA/RConn7
  OLTCA/RConn6 -- TransformerA/RConn6
  OLTCA/RConn5 -- TransformerA/RConn5
  OLTCA/RConn4 -- TransformerA/RConn4
  OLTCA/RConn3 -- TransformerA/RConn3
  OLTCA/RConn2 -- TransformerA/RConn2
  OLTCA/RConn1 -- TransformerA/RConn1
  Ground/LConn1 -- TransformerA/RConn23
  OLTCA/LConn1 -- a/RConn1
  Ground1/LConn1 -- TransformerB/RConn23
  OLTCA1/RConn7 -- TransformerB/RConn7
  OLTCA1/RConn17 -- TransformerB/RConn17
  OLTCA1/RConn21 -- TransformerB/RConn21
  OLTCA1/RConn15 -- TransformerB/RConn15
  OLTCA1/RConn14 -- TransformerB/RConn14
  OLTCA1/RConn3 -- TransformerB/RConn3
  OLTCA1/RConn9 -- TransformerB/RConn9
  OLTCA1/RConn13 -- TransformerB/RConn13
  OLTCA1/RConn8 -- TransformerB/RConn8
  OLTCA1/RConn1 -- TransformerB/RConn1
  OLTCA1/RConn16 -- TransformerB/RConn16
  OLTCA1/RConn12 -- TransformerB/RConn12
  OLTCA1/RConn4 -- TransformerB/RConn4
  OLTCA1/RConn5 -- TransformerB/RConn5
  OLTCA1/RConn2 -- TransformerB/RConn2
  OLTCA1/RConn10 -- TransformerB/RConn10
  OLTCA1/RConn6 -- TransformerB/RConn6
  OLTCA1/RConn20 -- TransformerB/RConn20
  OLTCA1/RConn22 -- TransformerB/RConn22
  OLTCA1/RConn18 -- TransformerB/RConn18
  OLTCA1/RConn19 -- TransformerB/RConn19
  OLTCA1/RConn11 -- TransformerB/RConn11
  Ground2/LConn1 -- TransformerC/RConn23
  OLTCA2/RConn7 -- TransformerC/RConn7
  OLTCA2/RConn17 -- TransformerC/RConn17
  OLTCA2/RConn21 -- TransformerC/RConn21
  OLTCA2/RConn15 -- TransformerC/RConn15
  OLTCA2/RConn14 -- TransformerC/RConn14
  OLTCA2/RConn3 -- TransformerC/RConn3
  OLTCA2/RConn9 -- TransformerC/RConn9
  OLTCA2/RConn13 -- TransformerC/RConn13
  OLTCA2/RConn8 -- TransformerC/RConn8
  OLTCA2/RConn1 -- TransformerC/RConn1
  OLTCA2/RConn16 -- TransformerC/RConn16
  OLTCA2/RConn12 -- TransformerC/RConn12
  OLTCA2/RConn4 -- TransformerC/RConn4
  OLTCA2/RConn5 -- TransformerC/RConn5
  OLTCA2/RConn2 -- TransformerC/RConn2
  OLTCA2/RConn10 -- TransformerC/RConn10
  OLTCA2/RConn6 -- TransformerC/RConn6
  OLTCA2/RConn20 -- TransformerC/RConn20
  OLTCA2/RConn22 -- TransformerC/RConn22
  OLTCA2/RConn18 -- TransformerC/RConn18
  OLTCA2/RConn19 -- TransformerC/RConn19
  OLTCA2/RConn11 -- TransformerC/RConn11
  OLTCA2/LConn1 -- c/RConn1
  OLTCA1/LConn1 -- b/RConn1
  TransformerA/LConn2 -- TransformerB/LConn1 -- B/RConn1
  TransformerB/LConn2 -- C/RConn1 -- TransformerC/LConn1
  TransformerC/LConn2 -- A/RConn1 -- TransformerA/LConn1

== system ANS_GFM_short_term/Synchronous Generator(GENTPJ) ==
  ve : Inport
  Pm : Inport  Port=2
  AVR+OEL+PSS : Subsystem  mask(AVR){ve0=Ve, uref=1.0, ifdlim=3.0618, L1=-20, L2=5, G=120, Ta=5, Tb=12.5, PSS_act=1, Kp=75, Tw=15, T1=0.22, T2=0.012, C=0.1}
      mask prompts: ve0 "Initialisierung Erregerspannung (ve0)"; uref "Referenzklemmenspannung (uref)"; ifdlim "max. Erregerstrom (ifdlim)"; L1 "Over-Excitation Limit (L1)"; L2 "AVR Limit (L2)"; G "Verstärkungsfaktor (G)"; Ta "AVR Zeitkonstante (Ta)"; Tb "AVR Zeitkonstante (Tb)"; PSS_act "PSS on/off (1/0)"; Kp "Verstärkungsfaktor PSS"; Tw "Wash-Out Filter (Tw)"; T1 "PSS Zeitkonstante (T1)"; T2 "PSS Zeitkonstante (T2)"; C "PSS Begrenzung"
      mask help: AVR
  Grid Interface : Subsystem
  Mechanical Equations : Subsystem
  Power calculation : Subsystem
  Rotor Equations : Subsystem
  Stator Equations : Subsystem
  Terminator : Terminator
  To Workspace1 : ToWorkspace  VariableName=psm  SampleTime=-1
      settings: Decimation=100
  To Workspace2 : ToWorkspace  VariableName=ifdsm  SampleTime=-1
      settings: Decimation=100
  a : PMIOPort  Side=Right
  b : PMIOPort  Port=2  Side=Right
  c : PMIOPort  Port=3  Side=Right
  delta : Outport
  wt : Outport  Port=2
  wires:
  Mechanical Equations/1(1+w) -> AVR+OEL+PSS/3(xspeed), Stator Equations/6(1+w), Power calculation/1(1+w)
  Stator Equations/2(Vqterm) -> Grid Interface/2(Vqterm), Power calculation/3(Vqterm)
  Power calculation/1(Te) -> To Workspace1/1, Mechanical Equations/2(Te)
  Rotor Equations/1(ifd) -> AVR+OEL+PSS/1(ie), To Workspace2/1
  Mechanical Equations/2(wt) -> Grid Interface/3(wt), wt/1
  Mechanical Equations/3(delta) -> delta/1
  Pm/1 -> Mechanical Equations/1(Pm)
  Rotor Equations/2(Edss) -> Stator Equations/3(Edss)
  Rotor Equations/3(Eqss) -> Stator Equations/4(Eqss)
  Grid Interface/1(id) -> Power calculation/4(Id), Stator Equations/1(Id), Rotor Equations/2(id)
  Grid Interface/2(iq) -> Power calculation/5(Iq), Stator Equations/2(Iq), Rotor Equations/3(iq)
  Grid Interface/4(|Uterm|) -> AVR+OEL+PSS/2(ut)
  ve/1 -> Terminator/1
  Stator Equations/1(Vdterm) -> Grid Interface/1(Vdterm), Power calculation/2(Vdterm)  "Eqs"
  Grid Interface/3(El) -> Stator Equations/5(E_l), Rotor Equations/4(El)
  AVR+OEL+PSS/1(ve) -> Rotor Equations/1(ve)
  connections:
  Grid Interface/RConn1 -- a/RConn1
  Grid Interface/RConn3 -- c/RConn1
  Grid Interface/RConn2 -- b/RConn1

== system ANS_GFM_short_term/Constant Current Load (EMT)/PLL ==
  Vabc : Inport
  Constant1 : Constant  Value=sqrt(2)*Pload/(sqrt(3)*Urms)
  Constant2 : Constant  Value=0
  Constant4 : Constant  Value=100*pi
  Cos : Trigonometry  Operator=cos
  Cos1 : Trigonometry
  Demux1 : Demux  Outputs=3
  Demux2 : Demux  Outputs=3
  Gain4 : Gain  Gain=Ki
  Gain5 : Gain  Gain=Kp
  Integrator2 : Integrator  InitialCondition=angle_load/180*pi-pi/2
  Integrator3 : Integrator
  Mux : Mux  Inputs=3
  Product : Product
  Product1 : Product
  Saturation1 : Saturate  UpperLimit=2*pi*55  LowerLimit=2*pi*45
  Sum2 : Sum  Inputs=|++
  Sum3 : Sum  Inputs=|++
  Sum4 : Sum  Inputs=-+
  Terminator : Terminator
  abc to Alpha-Beta-Zero : spsabctoAlphaBetaZeroLib/abc to Alpha-Beta-Zero
      settings: SourceProductBaseCode=PS
  delay : TransferFcn  Denominator=[Ts 1]
  dq0 to abc : spsdq0toabcLib/dq0 to abc  Alignment=Aligned with phase A axis
  Ia : Outport
  Ib : Outport  Port=2
  Ic : Outport  Port=3
  wires:
  Demux1/1 -> Ia/1
  Demux1/2 -> Ib/1
  Mux/1 -> dq0 to abc/1
  dq0 to abc/1 -> Demux1/1
  Demux1/3 -> Ic/1
  Constant2/1 -> Mux/2, Mux/3
  Constant1/1 -> Mux/1
  abc to Alpha-Beta-Zero/1 -> Demux2/1
  Sum2/1 -> Sum3/1
  Integrator3/1 -> Sum2/2
  Saturation1/1 -> Integrator2/1
  Gain5/1 -> Sum2/1
  Sum3/1 -> Saturation1/1
  Gain4/1 -> Integrator3/1
  Constant4/1 -> Sum3/2
  Product/1 -> Sum4/1
  Product1/1 -> Sum4/2
  Integrator2/1 -> Cos1/1, Cos/1, dq0 to abc/2
  Cos/1 -> Product1/2
  Cos1/1 -> Product/1
  Vabc/1 -> abc to Alpha-Beta-Zero/1
  Demux2/1 -> Product/2
  Demux2/2 -> Product1/1
  Sum4/1 -> delay/1
  delay/1 -> Gain4/1, Gain5/1
  Demux2/3 -> Terminator/1

== system ANS_GFM_short_term/GFM Converter/Converter (modified by S. Liemann) ==
  note: AC sources
  Vdq0 : Inport
  Pe_ac : Inport  Port=2
  Idc : Inport  Port=3
  wt : Inport  Port=4
  Divide : Product  Inputs=*/
  Gain12 : Gain  Gain=1/C_dc
  Gain13 : Gain  Gain=1/R_dc
  Gain8 : Gain  Gain=1/Vdc_n
  Integrator1 : Integrator  InitialCondition=Vdc_n
  Product5 : Product
  Subsystem1 : Subsystem
  Sum3 : Sum  Inputs=-+-
  dq0 to abc1 : spsdq0toabcLib/dq0 to abc  Alignment=90 degrees behind phase A axis
  a : PMIOPort  Side=Right
  b : PMIOPort  Port=2  Side=Right
  c : PMIOPort  Port=3  Side=Right
  Udc : Outport
  wires:
  Integrator1/1 -> Gain8/1, Divide/2, Udc/1, Gain13/1  "Udc"
  wt/1 -> dq0 to abc1/2
  Product5/1 -> dq0 to abc1/1
  Sum3/1 -> Gain12/1  "Ic"
  dq0 to abc1/1 -> Subsystem1/1(Vabc)
  Idc/1 -> Sum3/2
  Gain12/1 -> Integrator1/1
  Gain13/1 -> Sum3/3
  Vdq0/1 -> Product5/1
  Pe_ac/1 -> Divide/1
  Divide/1 -> Sum3/1
  Gain8/1 -> Product5/2
  connections:
  Subsystem1/RConn2 -- b/RConn1
  Subsystem1/RConn1 -- a/RConn1
  Subsystem1/RConn3 -- c/RConn1

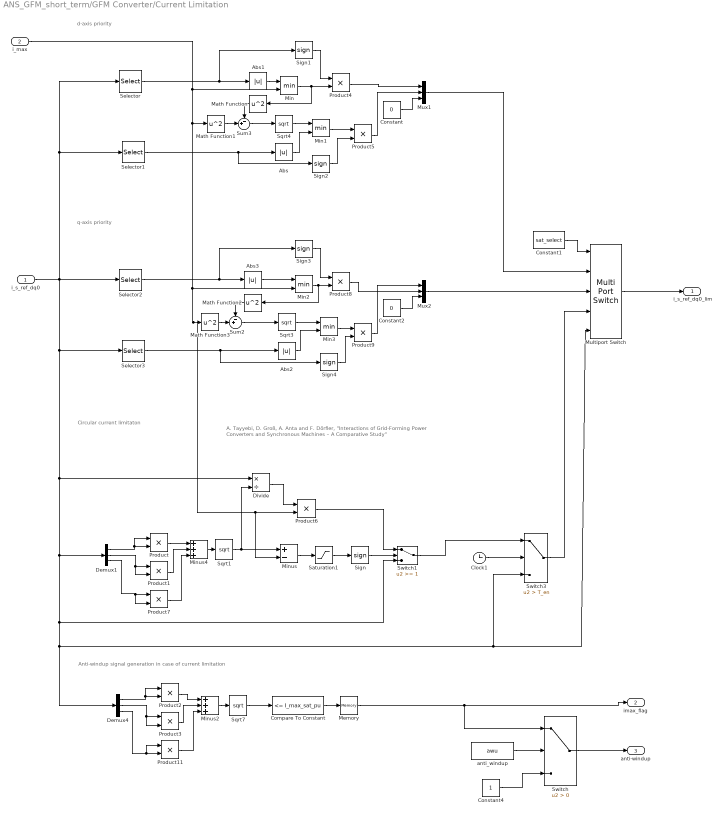
== system ANS_GFM_short_term/GFM Converter/Current Limitation ==
  note: Anti-windup signal generation in case of current limitation
  note: d-axis priority
  note: Circular current limitaton
  note: A. Tayyebi, D. Groß, A. Anta and F. Dörfler, "Interactions of Grid-Forming Power Converters and Synchronous Machines – A Comparative Study"
  note: q-axis priority
  i_s_ref_dq0 : Inport
  i_max : Inport  Port=2
  Abs{,1..3} (4 alike) : Abs
  Clock1 : Clock
  Compare To Constant : simulink/Logic and Bit Operations/Compare To Constant  relop=<=  const=I_max_sat_pu  OutDataTypeStr=boolean
  Constant : Constant  Value=0
  Constant1 : Constant  Value=sat_select
  Constant2 : Constant  Value=0
  Constant4 : Constant
  Demux1 : Demux  Outputs=3
  Demux4 : Demux  Outputs=3
  Divide : Product  Inputs=*/
  Math Function{,1..3} (4 alike) : Math  Operator=square  SaturateOnIntegerOverflow=on
  Memory : Memory  InitialCondition=1
  Min{,1..3} (4 alike) : MinMax  Inputs=2
  Minus : Sum  Inputs=+-
  Minus2 : Sum  Inputs=+++
  Minus4 : Sum  Inputs=+++
  Multiport Switch : MultiPortSwitch  Inputs=4
  Mux1 : Mux  Inputs=3
  Mux2 : Mux  Inputs=3
  Product{,1..3,6..7,11} (7 alike) : Product  RndMeth=Zero
  Product{4..5,8..9} (4 alike) : Product
  Saturation1 : Saturate  UpperLimit=inf  LowerLimit=0
  Selector : Selector  InputPortWidth=3  IndexOptions=Index vector (dialog)  Indices=[1 ]  OutputSizes=1
  Selector1 : Selector  InputPortWidth=3  IndexOptions=Index vector (dialog)  Indices=[2 ]  OutputSizes=1
  Selector2 : Selector  InputPortWidth=3  IndexOptions=Index vector (dialog)  Indices=[2 ]  OutputSizes=1
  Selector3 : Selector  InputPortWidth=3  IndexOptions=Index vector (dialog)  Indices=[1 ]  OutputSizes=1
  Sign{,1..4} (5 alike) : Signum
  Sqrt{1,3..4,7} (4 alike) : Sqrt  SaturateOnIntegerOverflow=on
  Sum2 : Sum  Inputs=-+|
  Sum3 : Sum  Inputs=-+|
  Switch : Switch  Criteria=u2 > Threshold
  Switch1 : Switch  Threshold=1
  Switch3 : Switch  Criteria=u2 > Threshold  Threshold=T_en
  anti_windup : Constant  Value=awu
  i_s_ref_dq0_lim : Outport  VectorParamsAs1DForOutWhenUnconnected=off
  imax_flag : Outport  Port=2
  anti-windup : Outport  Port=3
  wires:
  Demux1/3 -> Product7/2, Product7/1
  Product/1 -> Minus4/1
  Demux1/2 -> Product1/2, Product1/1
  Sqrt1/1 -> Minus/1, Divide/2
  Minus/1 -> Saturation1/1
  Demux1/1 -> Product/1, Product/2
  Product1/1 -> Minus4/2
  Minus4/1 -> Sqrt1/1
  Divide/1 -> Product6/1
  Saturation1/1 -> Sign/1
  Sign/1 -> Switch1/2
  Product7/1 -> Minus4/3
  Product6/1 -> Switch1/1
  Selector/1 -> Sign1/1, Abs1/1
  Sqrt4/1 -> Min1/1
  Sum3/1 -> Sqrt4/1
  Constant/1 -> Mux1/3
  Constant1/1 -> Multiport Switch/1
  Mux1/1 -> Multiport Switch/2
  Abs/1 -> Min1/2
  Selector1/1 -> Sign2/1, Abs/1
  Abs1/1 -> Min/1
  Sign1/1 -> Product4/1
  Min/1 -> Math Function/1, Product4/2
  Product4/1 -> Mux1/1
  Min1/1 -> Product5/1
  Product5/1 -> Mux1/2
  Sign2/1 -> Product5/2
  Sum2/1 -> Sqrt3/1
  Constant2/1 -> Mux2/3
  Product9/1 -> Mux2/1
  Selector3/1 -> Sign4/1, Abs2/1
  Abs2/1 -> Min3/2
  Sqrt3/1 -> Min3/1
  Selector2/1 -> Sign3/1, Abs3/1
  Abs3/1 -> Min2/1
  Product8/1 -> Mux2/2
  Sign4/1 -> Product9/2
  Min2/1 -> Math Function2/1, Product8/2
  Sign3/1 -> Product8/1
  Min3/1 -> Product9/1
  i_max/1 -> Math Function1/1, Minus/2, Product6/2, Math Function3/1, Min2/2, Min/2
  Mux2/1 -> Multiport Switch/3
  Math Function1/1 -> Sum3/2
  Math Function/1 -> Sum3/1
  Math Function3/1 -> Sum2/2
  Math Function2/1 -> Sum2/1
  Multiport Switch/1 -> i_s_ref_dq0_lim/1
  Minus2/1 -> Sqrt7/1
  Demux4/2 -> Product3/2, Product3/1
  Demux4/3 -> Product11/2, Product11/1
  Product3/1 -> Minus2/2
  Product11/1 -> Minus2/3
  Product2/1 -> Minus2/1
  Compare To Constant/1 -> Memory/1
  Demux4/1 -> Product2/1, Product2/2
  Sqrt7/1 -> Compare To Constant/1
  Switch/1 -> anti-windup/1
  Constant4/1 -> Switch/3
  anti_windup/1 -> Switch/2
  Switch1/1 -> Switch3/1
  Clock1/1 -> Switch3/2
  i_s_ref_dq0/1 -> Selector2/1, Selector1/1, Selector/1, Selector3/1, Switch3/3, Multiport Switch/5, Demux4/1, Switch1/3, Demux1/1, Divide/1
  Switch3/1 -> Multiport Switch/4
  Memory/1 -> imax_flag/1, Switch/1
